simulink model "ACFT"  (R2025a)
settings: Solver=ode1  StartTime=0.0  StopTime=200  FixedStep=0.01  RelTol=1e-3  EnableMultiTasking=on
model workspace (MAT data in the model file):
  op_trim2 : opcond.OperatingReport (value not decoded)
values from neighbouring files (symbols this model uses):
  alfaf_deg = -1.8    [initACFT_low.m]
  b = 21    [initACFT_low.m]
  c = 2.5    [initACFT_low.m]
  CD0 = 0.0230    (= 0.023)    [initACFT_low.m]
  CD_alpha = 0.1318    [initACFT_low.m]
  CD_elev = 0.0178    [initACFT_low.m]
  CL0 = 0.19    [initACFT_low.m]
  Cl_ail = -0.0516    [initACFT_low.m]
  CL_alpha = 6.1879    [initACFT_low.m]
  CL_AlphaDot = 1.93    [initACFT_low.m]
  Cl_beta = -0.1352    [initACFT_low.m]
  CL_elev = 0.4727    [initACFT_low.m]
  Cl_p = -0.45    [initACFT_low.m]
  CL_q = 4.66    [initACFT_low.m]
  Cl_r = 0.100    (= 0.1)    [initACFT_low.m]
  Cl_rud = 0.0289    [initACFT_low.m]
  Cm0 = 0.0133    [initACFT_low.m]
  Cm_alpha = -2.0168    [initACFT_low.m]
  Cm_AlphaDot = -6.76    [initACFT_low.m]
  Cm_elev = -1.6788    [initACFT_low.m]
  Cm_q = -36.3    [initACFT_low.m]
  Cn_ail = -6.3025e-4    (= -0.00063025)    [initACFT_low.m]
  Cn_beta = 0.1209    [initACFT_low.m]
  Cn_p = -0.114    [initACFT_low.m]
  Cn_r = -0.30    (= -0.3)    [initACFT_low.m]
  Cn_rud = -0.1020    (= -0.102)    [initACFT_low.m]
  CY_ail = 0    [initACFT_low.m]
  CY_beta = -1.1803    [initACFT_low.m]
  CY_p = 0.3    [initACFT_low.m]
  CY_r = 0.910    (= 0.91)    [initACFT_low.m]
  CY_rud = 0.4016    [initACFT_low.m]
  g = 9.80665    [initACFT_low.m]
  Inertia = [Ixx 0 -Ixz; 0 Iyy 0; -Ixz 0 Izz]    [initACFT_low.m]
  nrho = 0.75    [initACFT_low.m]
  nv = 0    [initACFT_low.m]
  rho_reference_kgpm3 = 1.225    [initACFT_low.m]
  S = 45    [initACFT_low.m]
  Tmax = 68000    [initACFT_low.m]
  V_reference_mps = 200    [initACFT_low.m]
  xf_m = -3.8    [initACFT_low.m]
  y_cg = 0    [initACFT_low.m]
  z_cg = -0.4    [initACFT_low.m]
  zf_m = -0.6    [initACFT_low.m]
undefined symbols (not defined in the file or in its folder): EqM
settings Model: PacingRate=0.890000  Creator=bruno  LastModifiedBy=best
settings SolverCC: AlgebraicLoopSolver=TrustRegion
settings DataIOCC: ExternalInput=getinputstruct(op_trim2)  InitialState=getstatestruct(op_trim2)  LoadExternalInput=on  LoadInitialState=on  ReturnWorkspaceOutputs=off
settings OptimizationCC: LifeSpan=inf
settings DebuggingCC: UnconnectedInputMsg=warning  UnconnectedOutputMsg=warning  UnconnectedLineMsg=warning  SFUnexpectedBacktrackingDiag=warning  SFNoUnconditionalDefaultTransitionDiag=warning  ArithmeticOperatorsInVariantConditions=warning
settings ModelReferenceCC: EnableRefExpFcnMdlSchedulingChecks=on
settings SFSimCC: SimUseLocalCustomCode=off  CustomCodeUndefinedFunction=UseInterfaceOnly
settings RTWCC: RTWUseLocalCustomCode=off  GPUComputeCapability=3.5
settings CodeAppCC: StateflowObjectComments=on
settings GRTTargetCC: TargetLangStandard=C89/C90 (ANSI)
settings ConfigComp: CovMetricSettings=dw  CovSaveCumulativeToWorkspaceVar=on  CovSaveSingleToWorkspaceVar=on  CovExternalEMLEnable=off

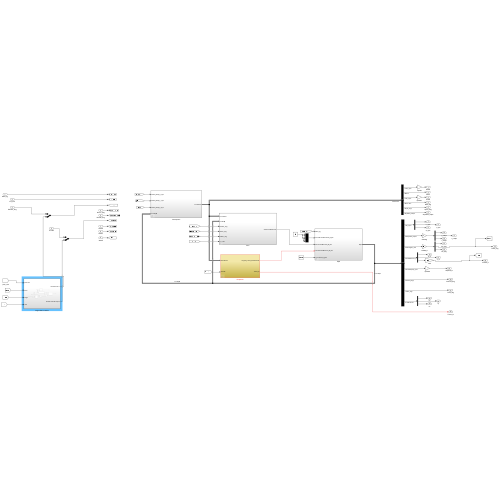
[thumbnail: Simulink's stored preview of the top-level diagram]
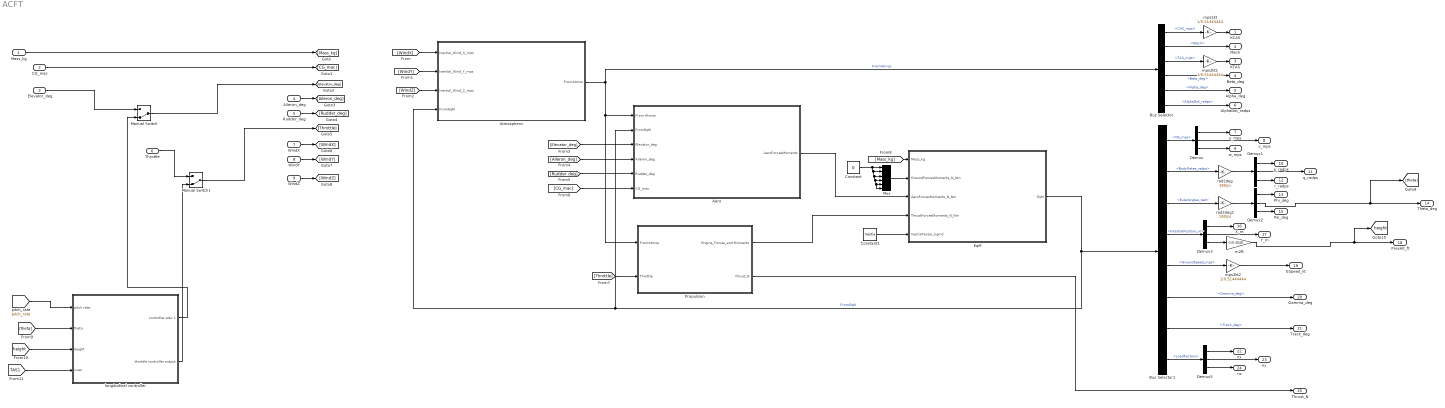
== system ACFT ==
  Mass_kg : Inport  OutDataTypeStr=double
  CG_mac : Inport  Port=2  OutDataTypeStr=double
  Elevator_deg : Inport  Port=3  OutDataTypeStr=double
  Aileron_deg : Inport  Port=4  OutDataTypeStr=double
  Rudder_deg : Inport  Port=5  OutDataTypeStr=double
  Throttle : Inport  Port=6  OutDataTypeStr=double
  WindX : Inport  Port=7  OutDataTypeStr=double
  WindY : Inport  Port=8  OutDataTypeStr=double
  WindZ : Inport  Port=9  OutDataTypeStr=double
  Aero : Subsystem  AncestorBlock=Aerodynamic/Aero
  Atmospheric : Subsystem  AncestorBlock=Atmospheric/Atmospheric
  Bus Selector : BusSelector  OutputSignals=CAS_mps,Mach,TAS_mps,Beta_deg,Alpha_deg,AlphaDot_radps
  Bus Selector1 : BusSelector  OutputSignals=VB_mps,BodyRates_radps,EulerAngles_rad,IntertialPosition_m,GroundSpeed_mps,Gamma_deg,Track_deg,LoadFactors
  Constant : Constant  Value=0  OutDataTypeStr=double
  Constant1 : Constant  Value=Inertia  OutDataTypeStr=double
  Demux{,1..3,5} (5 alike) : Demux  Outputs=3
  EqM : Subsystem  AncestorBlock=EqM/EqM
  Manual Switch : ManualSwitch  CurrentSetting=0
  Manual Switch1 : ManualSwitch  CurrentSetting=0
  Mux : Mux  Inputs=6
  Propulsion : Subsystem  AncestorBlock=Propulsion/Propulsion
  longitudinal controller : Subsystem
  m2ft : Gain  Gain=-1/0.3048
  mps2kt : Gain  Gain=1/0.51444444
  mps2kt1 : Gain  Gain=1/0.51444444
  mps2kt2 : Gain  Gain=1/0.51444444
  rad2deg : Gain  Gain=180/pi
  rad2deg1 : Gain  Gain=180/pi
  KCAS : Outport
  Mach : Outport  Port=2
  KTAS : Outport  Port=3
  Beta_deg : Outport  Port=4
  Alpha_deg : Outport  Port=5
  AlphaDot_radps : Outport  Port=6
  u_mps : Outport  Port=7
  v_mps : Outport  Port=8
  w_mps : Outport  Port=9
  p_radps : Outport  Port=10
  q_radps : Outport  Port=11
  r_radps : Outport  Port=12
  Phi_deg : Outport  Port=13
  Theta_deg : Outport  Port=14
  Psi_deg : Outport  Port=15
  X_m : Outport  Port=16
  Y_m : Outport  Port=17
  PresAlt_ft : Outport  Port=18
  GSpeed_kt : Outport  Port=19
  Gamma_deg : Outport  Port=20
  Track_deg : Outport  Port=21
  nx : Outport  Port=22
  ny : Outport  Port=23
  nz : Outport  Port=24
  Thrust_N : Outport  Port=25
  tag scope: height=global
  wires:
  Atmospheric/1(FromAtmos) -> Propulsion/1(FromAtmos), Aero/1(From Atmos), Bus Selector/1  "FromAtmos"
  Aero/1(AeroForcesMoments) -> EqM/3(AeroForcesMoments_N_Nm)
  Propulsion/1(Engine_Forces_and Moments) -> EqM/4(ThrustForcesMoments_N_Nm)
  EqM/1(EqM) -> Aero/2(FromEqM), Atmospheric/4(FromEqM), Bus Selector1/1  "FromEqM"
  Constant/1 -> Mux/6, Mux/5, Mux/4, Mux/3, Mux/2, Mux/1
  Mux/1 -> EqM/2(GroundForcesMoments_N_Nm)
  Constant1/1 -> EqM/5(InertiaTensor_kgm2)
  Mass_kg/1 -> [Mass_kg]
  CG_mac/1 -> [CG_mac]
  Elevator_deg/1 -> Manual Switch/1
  Aileron_deg/1 -> [Aileron_deg]
  Rudder_deg/1 -> [Rudder_deg]
  Throttle/1 -> Manual Switch1/1
  WindX/1 -> [WindX]
  WindY/1 -> [WindY]
  WindZ/1 -> [WindZ]
  [WindX] -> Atmospheric/1(Inertial_Wind_X_mps)
  [WindY] -> Atmospheric/2(Inertial_Wind_Y_mps)
  [WindZ] -> Atmospheric/3(Inertial_Wind_Z_mps)
  [Elevator_deg] -> Aero/3(Elevator_deg)
  [Aileron_deg] -> Aero/4(Aileron_deg)
  [Rudder_deg] -> Aero/5(Rudder_deg)
  [CG_mac] -> Aero/6(CG_mac)
  [Throttle] -> Propulsion/2(Throttle)
  [Mass_kg] -> EqM/1(Mass_kg)
  Propulsion/2(Thrust_N) -> Thrust_N/1
  Bus Selector/1 -> mps2kt/1  "<CAS_mps>"
  mps2kt/1 -> KCAS/1
  Bus Selector/2 -> Mach/1  "<Mach>"
  Bus Selector/3 -> mps2kt1/1  "<TAS_mps>"
  mps2kt1/1 -> KTAS/1
  Bus Selector/4 -> Beta_deg/1  "<Beta_deg>"
  Bus Selector/5 -> Alpha_deg/1  "<Alpha_deg>"
  Bus Selector/6 -> AlphaDot_radps/1  "<AlphaDot_radps>"
  Bus Selector1/1 -> Demux/1  "<VB_mps>"
  Demux/1 -> u_mps/1
  Demux/2 -> v_mps/1
  Demux/3 -> w_mps/1
  Bus Selector1/2 -> rad2deg/1  "<BodyRates_radps>"
  Demux1/1 -> p_radps/1
  Demux1/2 -> q_radps/1
  Demux1/3 -> r_radps/1
  Bus Selector1/3 -> rad2deg1/1  "<EulerAngles_rad>"
  Demux2/1 -> Phi_deg/1
  Demux2/2 -> [theta], Theta_deg/1
  Demux2/3 -> Psi_deg/1
  rad2deg/1 -> Demux1/1
  rad2deg1/1 -> Demux2/1
  Bus Selector1/4 -> Demux3/1  "<IntertialPosition_m>"
  Demux3/1 -> X_m/1
  Demux3/2 -> Y_m/1
  Demux3/3 -> m2ft/1
  m2ft/1 -> [height], PresAlt_ft/1
  Bus Selector1/5 -> mps2kt2/1  "<GroundSpeed_mps>"
  mps2kt2/1 -> GSpeed_kt/1
  Bus Selector1/6 -> Gamma_deg/1  "<Gamma_deg>"
  Bus Selector1/7 -> Track_deg/1  "<Track_deg>"
  Bus Selector1/8 -> Demux5/1  "<LoadFactors>"
  Demux5/1 -> nx/1
  Demux5/2 -> ny/1
  Demux5/3 -> nz/1
  [pitch_rate] -> longitudinal controller/1(pitch rate)
  [theta] -> longitudinal controller/2(theta)
  [height] -> longitudinal controller/3(height)
  [TAS1] -> longitudinal controller/4(vcas)
  longitudinal controller/1(controller elev 1) -> Manual Switch/2
  Manual Switch/1 -> [Elevator_deg]
  longitudinal controller/2(throttle controller output) -> Manual Switch1/2
  Manual Switch1/1 -> [Throttle]

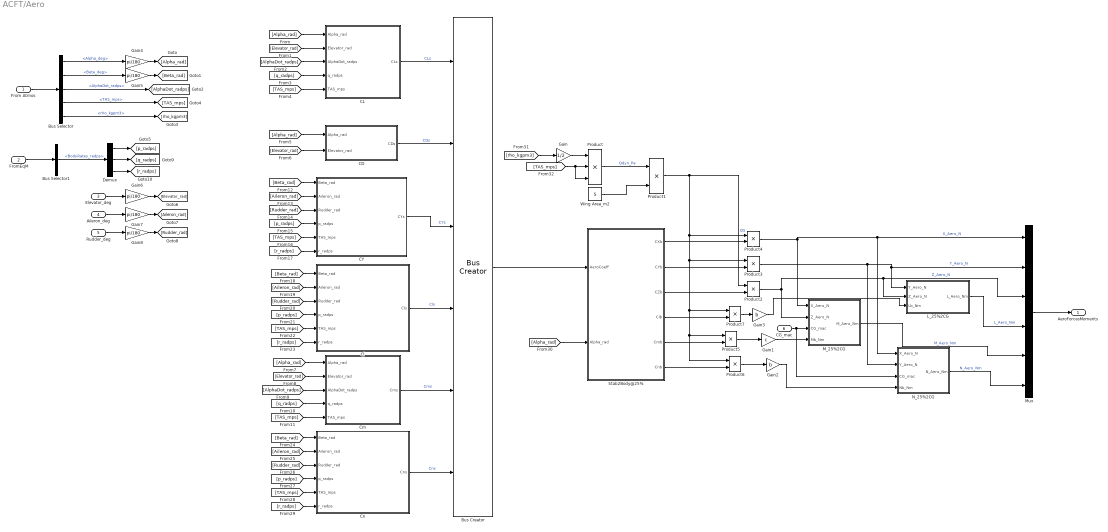
== system ACFT/Aero ==
  From Atmos : Inport
  FromEqM : Inport  Port=2
  Elevator_deg : Inport  Port=3
  Aileron_deg : Inport  Port=4
  Rudder_deg : Inport  Port=5
  CG_mac : Inport  Port=6
  Bus Creator : BusCreator  Inputs=6
  Bus Selector : BusSelector  OutputSignals=Alpha_deg,Beta_deg,AlphaDot_radps,TAS_mps,rho_kgpm3
  Bus Selector1 : BusSelector  OutputSignals=BodyRates_radps
  CD : Subsystem
  CL : Subsystem
  CY : Subsystem
  Cl : Subsystem
  Cm : Subsystem
  Cn : Subsystem
  Demux : Demux  Outputs=3
  Gain : Gain  Gain=1/2
  Gain1 : Gain  Gain=c
  Gain2 : Gain  Gain=b
  Gain3 : Gain  Gain=b
  Gain{4..8} (5 alike) : Gain  Gain=pi/180
  L_25%2CG : Subsystem
  M_25%2CG : Subsystem
  Mux : Mux  Inputs=6
  N_25%2CG : Subsystem
  Product : Product  Inputs=3
  Product{1..7} (7 alike) : Product
  Stab2Body@25% : Subsystem
  Wing Area_m2 : Constant  Value=S
  AeroForcesMoments : Outport
  wires:
  Bus Selector/5 -> [rho_kgpm3]  "<rho_kgpm3>"
  Bus Selector/4 -> [TAS_mps]  "<TAS_mps>"
  N_25%2CG/1(N_Aero_Nm) -> Mux/6  "N_Aero_Nm"
  Product/1 -> Product1/1  "Qdyn_Pa"
  [Aileron_rad] -> Cn/2(Aileron_rad)
  [p_radps] -> Cn/4(p_radps)
  Product5/1 -> Gain1/1
  [q_radps] -> Cm/4(q_radps)
  [AlphaDot_radps] -> Cm/3(AlphaDot_radps)
  CG_mac/1 -> M_25%2CG/3(CG_mac), N_25%2CG/3(CG_mac)
  Product4/1 -> M_25%2CG/1(X_Aero_N), N_25%2CG/1(X_Aero_N), Mux/1  "X_Aero_N"
  [Alpha_rad] -> Stab2Body@25%/2(Alpha_rad)
  Cn/1(Cns) -> Bus Creator/6  "Cns"
  [TAS_mps] -> Cl/5(TAS_mps)
  CL/1(CLs) -> Bus Creator/1  "CLs"
  L_25%2CG/1(L_Aero_Nm) -> Mux/4  "L_Aero_Nm"
  [Aileron_rad] -> CY/2(Aileron_rad)
  Cm/1(Cms) -> Bus Creator/5  "Cms"
  Gain3/1 -> L_25%2CG/3(Lb_Nm)
  Product6/1 -> Gain2/1
  M_25%2CG/1(M_Aero_Nm) -> Mux/5  "M_Aero_Nm"
  CY/1(CYs) -> Bus Creator/3  "CYs"
  [Rudder_rad] -> Cl/3(Rudder_rad)
  [r_radps] -> Cl/6(r_radps)
  Stab2Body@25%/5(Cmb) -> Product5/2
  Gain/1 -> Product/1
  [TAS_mps] -> Cm/5(TAS_mps)
  Stab2Body@25%/3(CZb) -> Product2/2
  [TAS_mps] -> Product/2, Product/3
  [TAS_mps] -> CY/5(TAS_mps)
  Product3/1 -> N_25%2CG/2(Y_Aero_N), L_25%2CG/1(Y_Aero_N), Mux/2  "Y_Aero_N"
  [Aileron_rad] -> Cl/2(Aileron_rad)
  [rho_kgpm3] -> Gain/1
  Product7/1 -> Gain3/1
  Stab2Body@25%/4(Clb) -> Product7/2
  [Rudder_rad] -> Cn/3(Rudder_rad)
  Bus Creator/1 -> Stab2Body@25%/1(AeroCoeff)
  [r_radps] -> Cn/6(r_radps)
  Product2/1 -> M_25%2CG/2(Z_Aero_N), L_25%2CG/2(Z_Aero_N), Mux/3  "Z_Aero_N"
  CD/1(CDs) -> Bus Creator/2  "CDs"
  [TAS_mps] -> Cn/5(TAS_mps)
  Stab2Body@25%/6(Cnb) -> Product6/2
  Product1/1 -> Product4/1, Product5/1, Product6/1, Product7/1, Product3/1, Product2/1  "QS"
  Gain2/1 -> N_25%2CG/4(Nb_Nm)
  Stab2Body@25%/1(CXb) -> Product4/2
  Cl/1(Cls) -> Bus Creator/4  "Cls"
  Wing Area_m2/1 -> Product1/2
  [r_radps] -> CY/6(r_radps)
  [Beta_rad] -> CY/1(Beta_rad)
  [Rudder_rad] -> CY/3(Rudder_rad)
  [Beta_rad] -> Cn/1(Beta_rad)
  [Beta_rad] -> Cl/1(Beta_rad)
  Gain1/1 -> M_25%2CG/4(Mb_Nm)
  [p_radps] -> Cl/4(p_radps)
  Stab2Body@25%/2(CYb) -> Product3/2
  [p_radps] -> CY/4(p_radps)
  Mux/1 -> AeroForcesMoments/1
  Gain5/1 -> [Beta_rad]
  Gain4/1 -> [Alpha_rad]
  Rudder_deg/1 -> Gain8/1
  Bus Selector/3 -> [AlphaDot_radps]  "<AlphaDot_radps>"
  [Elevator_rad] -> Cm/2(Elevator_rad)
  [Alpha_rad] -> Cm/1(Alpha_rad)
  [Elevator_rad] -> CL/2(Elevator_rad)
  Elevator_deg/1 -> Gain6/1
  [Alpha_rad] -> CL/1(Alpha_rad)
  [Elevator_rad] -> CD/2(Elevator_rad)
  Gain8/1 -> [Rudder_rad]
  [Alpha_rad] -> CD/1(Alpha_rad)
  [q_radps] -> CL/4(q_radps)
  Bus Selector/2 -> Gain5/1  "<Beta_deg>"
  Gain7/1 -> [Aileron_rad]
  Aileron_deg/1 -> Gain7/1
  Demux/2 -> [q_radps]
  Demux/1 -> [p_radps]
  Gain6/1 -> [Elevator_rad]
  Demux/3 -> [r_radps]
  [TAS_mps] -> CL/5(TAS_mps)
  [AlphaDot_radps] -> CL/3(AlphaDot_radps)
  From Atmos/1 -> Bus Selector/1
  Bus Selector/1 -> Gain4/1  "<Alpha_deg>"
  FromEqM/1 -> Bus Selector1/1
  Bus Selector1/1 -> Demux/1  "<BodyRates_radps>"

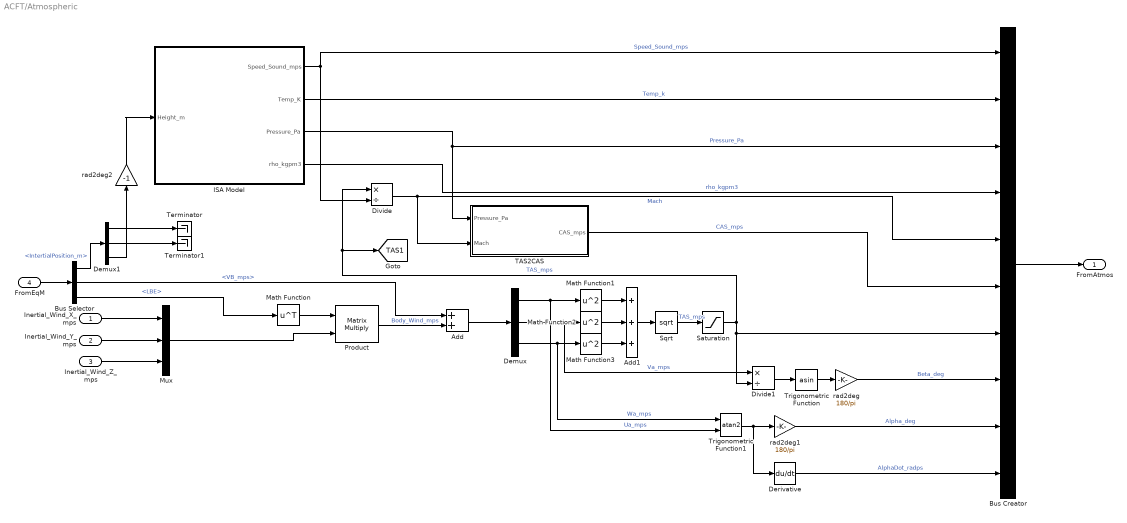
== system ACFT/Atmospheric ==
  Inertial_Wind_X_mps : Inport
  Inertial_Wind_Y_mps : Inport  Port=2
  Inertial_Wind_Z_mps : Inport  Port=3
  FromEqM : Inport  Port=4
  Add : Sum
  Add1 : Sum  Inputs=+++
  Bus Creator : BusCreator  Inputs=10
  Bus Selector : BusSelector  OutputSignals=IntertialPosition_m,VB_mps,LBE
  Demux : Demux  Outputs=3
  Demux1 : Demux  Outputs=3
  Derivative : Derivative
  Divide : Product  Inputs=*/
  Divide1 : Product  Inputs=*/
  ISA Model : Subsystem
  Math Function : Math  Operator=transpose  SignedPower=on
  Math Function1 : Math  Operator=square  SignedPower=on
  Math Function2 : Math  Operator=square  SignedPower=on
  Math Function3 : Math  Operator=square  SignedPower=on
  Mux : Mux  Inputs=3
  Product : Product  Multiplication=Matrix(*)
  Saturation : Saturate  UpperLimit=inf  LowerLimit=1
  Sqrt : Sqrt
  TAS2CAS : Subsystem
  Terminator : Terminator
  Terminator1 : Terminator
  Trigonometric Function : Trigonometry  Operator=asin
  Trigonometric Function1 : Trigonometry  Operator=atan2
  rad2deg : Gain  Gain=180/pi
  rad2deg1 : Gain  Gain=180/pi
  rad2deg2 : Gain  Gain=-1
  FromAtmos : Outport
  tag scope: TAS1=global
  wires:
  rad2deg/1 -> Bus Creator/8  "Beta_deg"
  Math Function3/1 -> Add1/3
  Add1/1 -> Sqrt/1
  Math Function1/1 -> Add1/1
  Demux/2 -> Math Function2/1, Divide1/1  "Va_mps"
  Demux/3 -> Math Function3/1, Trigonometric Function1/1  "Wa_mps"
  Divide1/1 -> Trigonometric Function/1
  Trigonometric Function/1 -> rad2deg/1
  Math Function2/1 -> Add1/2
  Demux/1 -> Math Function1/1, Trigonometric Function1/2  "Ua_mps"
  Add/1 -> Demux/1
  Demux1/3 -> rad2deg2/1
  TAS2CAS/1(CAS_mps) -> Bus Creator/6  "CAS_mps"
  Product/1 -> Add/2  "Body_Wind_mps"
  Mux/1 -> Product/2
  Math Function/1 -> Product/1
  Inertial_Wind_Z_mps/1 -> Mux/3
  Sqrt/1 -> Saturation/1  "TAS_mps"
  FromEqM/1 -> Bus Selector/1
  Divide/1 -> Bus Creator/5, TAS2CAS/2(Mach)  "Mach"
  ISA Model/3(Pressure_Pa) -> Bus Creator/3, TAS2CAS/1(Pressure_Pa)  "Pressure_Pa"
  Inertial_Wind_X_mps/1 -> Mux/1
  ISA Model/2(Temp_K) -> Bus Creator/2  "Temp_k"
  Inertial_Wind_Y_mps/1 -> Mux/2
  ISA Model/1(Speed_Sound_mps) -> Divide/2, Bus Creator/1  "Speed_Sound_mps"
  ISA Model/4(rho_kgpm3) -> Bus Creator/4  "rho_kgpm3"
  rad2deg1/1 -> Bus Creator/9  "Alpha_deg"
  Bus Creator/1 -> FromAtmos/1
  Trigonometric Function1/1 -> rad2deg1/1, Derivative/1
  Derivative/1 -> Bus Creator/10  "AlphaDot_radps"
  Bus Selector/3 -> Math Function/1  "<LBE>"
  Bus Selector/2 -> Add/1  "<VB_mps>"
  Bus Selector/1 -> Demux1/1  "<IntertialPosition_m>"
  Demux1/1 -> Terminator/1
  Demux1/2 -> Terminator1/1
  rad2deg2/1 -> ISA Model/1("Height_m ")
  Saturation/1 -> [TAS1], Divide/1, Bus Creator/7, Divide1/2  "TAS_mps"

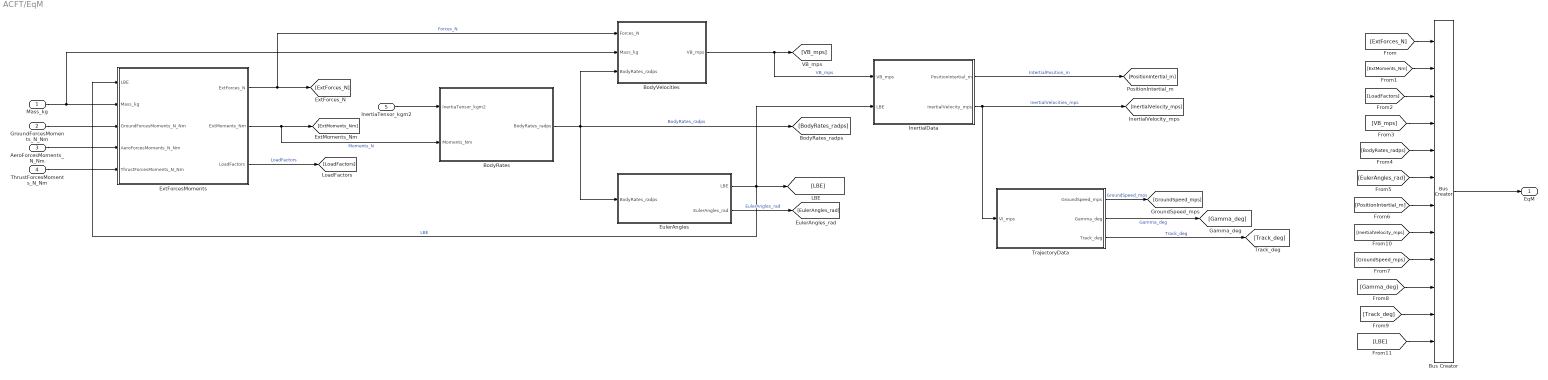
== system ACFT/EqM ==
  Mass_kg : Inport
  GroundForcesMoments_N_Nm : Inport  Port=2
  AeroForcesMoments_N_Nm : Inport  Port=3
  ThrustForcesMoments_N_Nm : Inport  Port=4
  InertiaTensor_kgm2 : Inport  Port=5
  BodyRates : Subsystem
  BodyVelocities : Subsystem
  Bus Creator : BusCreator  Inputs=12
  EulerAngles : Subsystem
  ExtForcesMoments : Subsystem
  InertialData : Subsystem
  TrajectoryData : Subsystem
  EqM : Outport
  wires:
  [PositionIntertial_m] -> Bus Creator/7
  [EulerAngles_rad] -> Bus Creator/6
  [BodyRates_radps] -> Bus Creator/5
  [VB_mps] -> Bus Creator/4
  [ExtForces_N] -> Bus Creator/1
  Bus Creator/1 -> EqM/1
  [Track_deg] -> Bus Creator/11
  [ExtMoments_Nm] -> Bus Creator/2
  [Gamma_deg] -> Bus Creator/10
  [GroundSpeed_mps] -> Bus Creator/9
  TrajectoryData/1(GroundSpeed_mps) -> [GroundSpeed_mps]  "GroundSpeed_mps"
  EulerAngles/2(EulerAngles_rad) -> [EulerAngles_rad]  "EulerAngles_rad"
  TrajectoryData/3(Track_deg) -> [Track_deg]  "Track_deg"
  TrajectoryData/2(Gamma_deg) -> [Gamma_deg]  "Gamma_deg"
  AeroForcesMoments_N_Nm/1 -> ExtForcesMoments/4(AeroForcesMoments_N_Nm)
  ExtForcesMoments/3(LoadFactors) -> [LoadFactors]  "LoadFactors"
  Mass_kg/1 -> ExtForcesMoments/2(Mass_kg), BodyVelocities/2(Mass_kg)
  ExtForcesMoments/1(ExtForces_N) -> BodyVelocities/1(Forces_N), [ExtForces_N]  "Forces_N"
  BodyVelocities/1(VB_mps) -> InertialData/1(VB_mps), [VB_mps]  "VB_mps"
  EulerAngles/1(LBE) -> [LBE], ExtForcesMoments/1(LBE), InertialData/2(LBE)  "LBE"
  GroundForcesMoments_N_Nm/1 -> ExtForcesMoments/3(GroundForcesMoments_N_Nm)
  ThrustForcesMoments_N_Nm/1 -> ExtForcesMoments/5(ThrustForcesMoments_N_Nm)
  BodyRates/1(BodyRates_radps) -> BodyVelocities/3(BodyRates_radps), EulerAngles/1(BodyRates_radps), [BodyRates_radps]  "BodyRates_radps"
  InertiaTensor_kgm2/1 -> BodyRates/1(InertiaTensor_kgm2)
  ExtForcesMoments/2(ExtMoments_Nm) -> BodyRates/2(Moments_Nm), [ExtMoments_Nm]  "Moments_N"
  [InertialVelocity_mps] -> Bus Creator/8
  [LoadFactors] -> Bus Creator/3
  InertialData/2(InertialVelocity_mps) -> TrajectoryData/1(VI_mps), [InertialVelocity_mps]  "InertialVelocities_mps"
  InertialData/1(PositionIntertial_m) -> [PositionIntertial_m]  "IntertialPosition_m"
  [LBE] -> Bus Creator/12

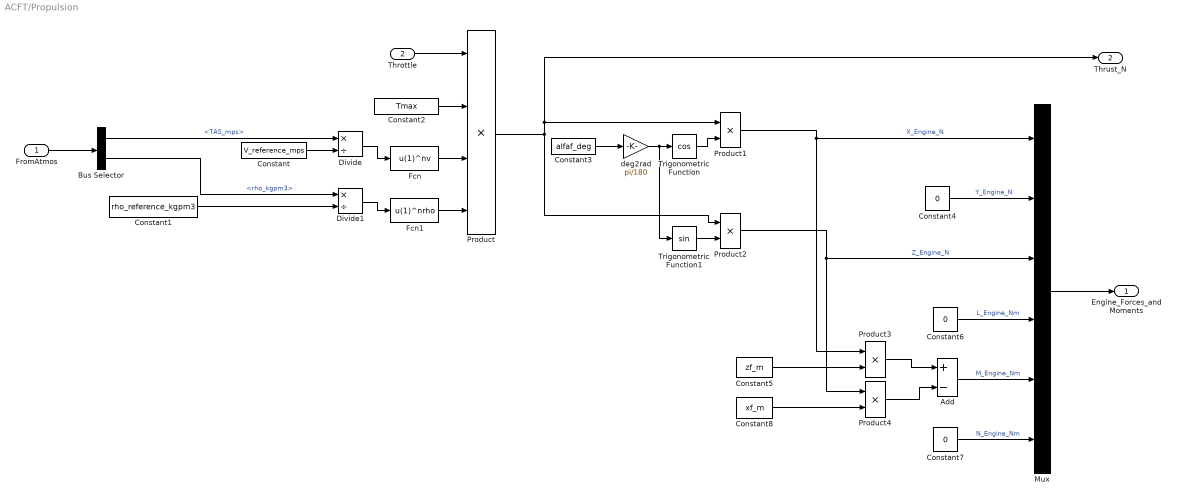
== system ACFT/Propulsion ==
  FromAtmos : Inport
  Throttle : Inport  Port=2
  Add : Sum  Inputs=+-
  Bus Selector : BusSelector  OutputSignals=TAS_mps,rho_kgpm3
  Constant : Constant  Value=V_reference_mps
  Constant1 : Constant  Value=rho_reference_kgpm3
  Constant2 : Constant  Value=Tmax
  Constant3 : Constant  Value=alfaf_deg
  Constant4 : Constant  Value=0
  Constant5 : Constant  Value=zf_m
  Constant6 : Constant  Value=0
  Constant7 : Constant  Value=0
  Constant8 : Constant  Value=xf_m
  Divide : Product  Inputs=*/
  Divide1 : Product  Inputs=*/
  Fcn : Fcn  Expr=u(1)^nv
  Fcn1 : Fcn  Expr=u(1)^nrho
  Mux : Mux  Inputs=6
  Product : Product  Inputs=4
  Product{1..4} (4 alike) : Product
  Trigonometric Function : Trigonometry  Operator=cos
  Trigonometric Function1 : Trigonometry
  deg2rad : Gain  Gain=pi/180
  Engine_Forces_and Moments : Outport
  Thrust_N : Outport  Port=2
  wires:
  Bus Selector/1 -> Divide/1  "<TAS_mps>"
  Add/1 -> Mux/5  "M_Engine_Nm"
  Constant8/1 -> Product4/2
  Constant4/1 -> Mux/2  "Y_Engine_N"
  Trigonometric Function/1 -> Product1/2
  Product1/1 -> Product3/1, Mux/1  "X_Engine_N"
  deg2rad/1 -> Trigonometric Function/1, Trigonometric Function1/1
  Product/1 -> Product1/1, Thrust_N/1, Product2/1
  Mux/1 -> Engine_Forces_and Moments/1
  Product2/1 -> Product4/1, Mux/3  "Z_Engine_N"
  FromAtmos/1 -> Bus Selector/1
  Divide/1 -> Fcn/1
  Constant2/1 -> Product/2
  Fcn/1 -> Product/3
  Bus Selector/2 -> Divide1/1  "<rho_kgpm3>"
  Constant7/1 -> Mux/6  "N_Engine_Nm"
  Fcn1/1 -> Product/4
  Constant6/1 -> Mux/4  "L_Engine_Nm"
  Product4/1 -> Add/2
  Constant3/1 -> deg2rad/1
  Constant5/1 -> Product3/2
  Divide1/1 -> Fcn1/1
  Constant1/1 -> Divide1/2
  Product3/1 -> Add/1
  Constant/1 -> Divide/2
  Throttle/1 -> Product/1
  Trigonometric Function1/1 -> Product2/2

== system ACFT/longitudinal controller ==
  pitch rate : Inport
  theta : Inport  Port=2
  height : Inport  Port=3
  vcas : Inport  Port=4
  Manual Switch : ManualSwitch  CurrentSetting=0
  Manual Switch1 : ManualSwitch  CurrentSetting=0
  Scope : Scope
      settings: ActiveDisplayYMinimum=-90.042313171294722  ActiveDisplayYMaximum=5604.3230575838888
  airspeed_pitchcontrol : Subsystem
  altitude_hold : Subsystem
  commande_pitch : Constant  Value=3
  commanded airspeed : Constant  Value=100
  commanded height : Constant  Value=500
  pitch_attitude_controller : Subsystem
  throttle_control : Subsystem
  controller elev 1 : Outport
  throttle controller output : Outport  Port=2
  wires:
  vcas/1 -> throttle_control/1(vcas), airspeed_pitchcontrol/1(vcas)
  height/1 -> Scope/1, altitude_hold/1(height)
  altitude_hold/1(commanded_pitch) -> Manual Switch/2
  commanded height/1 -> altitude_hold/2(commanded_altitude)
  throttle_control/1(throttle controller output) -> throttle controller output/1
  commanded airspeed/1 -> throttle_control/2(commanded_airspeed), airspeed_pitchcontrol/2(commanded_airspeed)
  commande_pitch/1 -> Manual Switch/1
  airspeed_pitchcontrol/1(commanded_pitch) -> Manual Switch1/1
  pitch rate/1 -> pitch_attitude_controller/1(pitch rate)
  theta/1 -> pitch_attitude_controller/2(theta)
  Manual Switch1/1 -> pitch_attitude_controller/3(commanded_pitch)
  pitch_attitude_controller/1(controller elev 1) -> controller elev 1/1
  Manual Switch/1 -> Manual Switch1/2

== system ACFT/Aero/CD ==
  Alpha_rad : Inport
  Elevator_rad : Inport  Port=2
  Abs : Abs  SaturateOnIntegerOverflow=off
  Abs1 : Abs  SaturateOnIntegerOverflow=off
  Add : Sum  Inputs=+++
  Constant : Constant  Value=CD0
  Gain : Gain  Gain=CD_alpha
  Gain1 : Gain  Gain=CD_elev
  CDs : Outport
  wires:
  Gain/1 -> Add/2
  Alpha_rad/1 -> Abs/1
  Add/1 -> CDs/1
  Elevator_rad/1 -> Abs1/1
  Constant/1 -> Add/1
  Abs/1 -> Gain/1
  Gain1/1 -> Add/3
  Abs1/1 -> Gain1/1

== system ACFT/Aero/CL ==
  Alpha_rad : Inport
  Elevator_rad : Inport  Port=2
  AlphaDot_radps : Inport  Port=3
  q_radps : Inport  Port=4
  TAS_mps : Inport  Port=5
  Add : Sum  Inputs=+++++
  Constant : Constant  Value=CL0
  Divide : Product  Inputs=*/
  Divide1 : Product  Inputs=*/
  Gain : Gain  Gain=CL_alpha
  Gain1 : Gain  Gain=CL_elev
  Gain2 : Gain  Gain=CL_AlphaDot
  Gain3 : Gain  Gain=CL_q
  Gain4 : Gain  Gain=c
  Gain5 : Gain  Gain=2
  Gain6 : Gain  Gain=c
  Gain7 : Gain  Gain=2
  CLs : Outport
  wires:
  AlphaDot_radps/1 -> Gain2/1
  Elevator_rad/1 -> Gain1/1
  q_radps/1 -> Gain3/1
  Gain/1 -> Add/2
  Constant/1 -> Add/1
  Gain1/1 -> Add/3
  Alpha_rad/1 -> Gain/1
  Add/1 -> CLs/1
  Gain3/1 -> Gain4/1
  Gain4/1 -> Divide/1
  TAS_mps/1 -> Gain7/1, Gain5/1
  Gain5/1 -> Divide/2
  Divide/1 -> Add/5
  Gain2/1 -> Gain6/1
  Gain6/1 -> Divide1/1
  Gain7/1 -> Divide1/2
  Divide1/1 -> Add/4

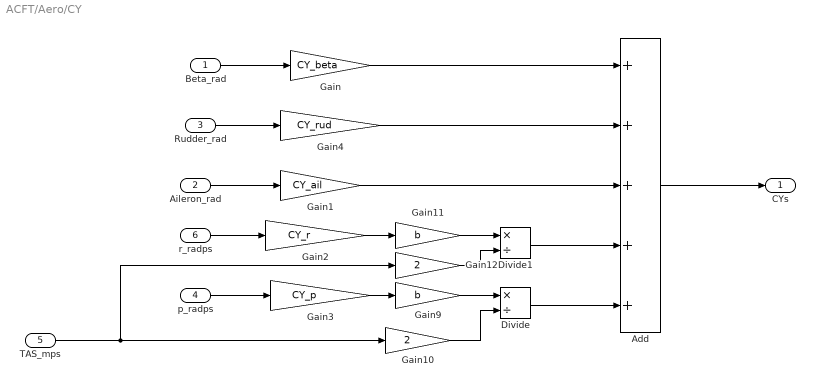
== system ACFT/Aero/CY ==
  Beta_rad : Inport
  Aileron_rad : Inport  Port=2
  Rudder_rad : Inport  Port=3
  p_radps : Inport  Port=4
  TAS_mps : Inport  Port=5
  r_radps : Inport  Port=6
  Add : Sum  Inputs=+++++
  Divide : Product  Inputs=*/
  Divide1 : Product  Inputs=*/
  Gain : Gain  Gain=CY_beta
  Gain1 : Gain  Gain=CY_ail
  Gain10 : Gain  Gain=2
  Gain11 : Gain  Gain=b
  Gain12 : Gain  Gain=2
  Gain2 : Gain  Gain=CY_r
  Gain3 : Gain  Gain=CY_p
  Gain4 : Gain  Gain=CY_rud
  Gain9 : Gain  Gain=b
  CYs : Outport
  wires:
  Aileron_rad/1 -> Gain1/1
  p_radps/1 -> Gain3/1
  Gain3/1 -> Gain9/1
  Beta_rad/1 -> Gain/1
  TAS_mps/1 -> Gain12/1, Gain10/1
  Divide/1 -> Add/5
  Add/1 -> CYs/1
  Gain11/1 -> Divide1/1
  Gain12/1 -> Divide1/2
  Gain10/1 -> Divide/2
  Gain1/1 -> Add/3
  Gain9/1 -> Divide/1
  Gain2/1 -> Gain11/1
  Divide1/1 -> Add/4
  Gain/1 -> Add/1
  Rudder_rad/1 -> Gain4/1
  Gain4/1 -> Add/2
  r_radps/1 -> Gain2/1

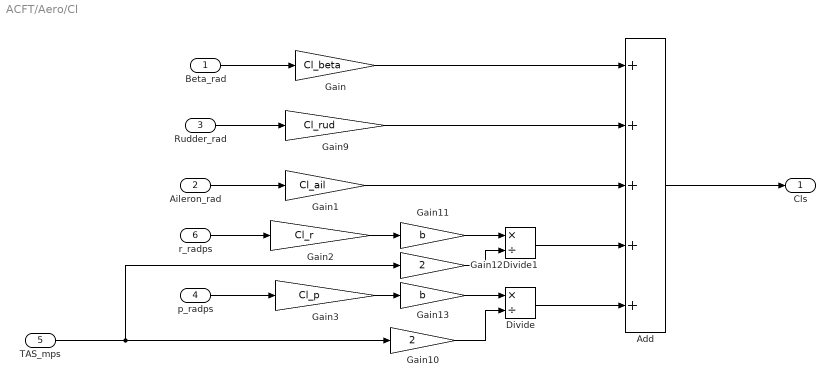
== system ACFT/Aero/Cl ==
  Beta_rad : Inport
  Aileron_rad : Inport  Port=2
  Rudder_rad : Inport  Port=3
  p_radps : Inport  Port=4
  TAS_mps : Inport  Port=5
  r_radps : Inport  Port=6
  Add : Sum  Inputs=+++++
  Divide : Product  Inputs=*/
  Divide1 : Product  Inputs=*/
  Gain : Gain  Gain=Cl_beta
  Gain1 : Gain  Gain=Cl_ail
  Gain10 : Gain  Gain=2
  Gain11 : Gain  Gain=b
  Gain12 : Gain  Gain=2
  Gain13 : Gain  Gain=b
  Gain2 : Gain  Gain=Cl_r
  Gain3 : Gain  Gain=Cl_p
  Gain9 : Gain  Gain=Cl_rud
  Cls : Outport
  wires:
  Aileron_rad/1 -> Gain1/1
  p_radps/1 -> Gain3/1
  Gain3/1 -> Gain13/1
  Beta_rad/1 -> Gain/1
  TAS_mps/1 -> Gain12/1, Gain10/1
  r_radps/1 -> Gain2/1
  Gain1/1 -> Add/3
  Gain11/1 -> Divide1/1
  Gain/1 -> Add/1
  Add/1 -> Cls/1
  Rudder_rad/1 -> Gain9/1
  Gain10/1 -> Divide/2
  Gain12/1 -> Divide1/2
  Gain9/1 -> Add/2
  Gain2/1 -> Gain11/1
  Divide1/1 -> Add/4
  Divide/1 -> Add/5
  Gain13/1 -> Divide/1

== system ACFT/Aero/Cm ==
  Alpha_rad : Inport
  Elevator_rad : Inport  Port=2
  AlphaDot_radps : Inport  Port=3
  q_radps : Inport  Port=4
  TAS_mps : Inport  Port=5
  Add : Sum  Inputs=+++++
  Constant : Constant  Value=Cm0
  Divide : Product  Inputs=*/
  Divide1 : Product  Inputs=*/
  Gain : Gain  Gain=Cm_alpha
  Gain1 : Gain  Gain=Cm_elev
  Gain10 : Gain  Gain=2
  Gain11 : Gain  Gain=c
  Gain12 : Gain  Gain=2
  Gain2 : Gain  Gain=Cm_AlphaDot
  Gain3 : Gain  Gain=Cm_q
  Gain9 : Gain  Gain=c
  Cms : Outport
  wires:
  AlphaDot_radps/1 -> Gain2/1
  Elevator_rad/1 -> Gain1/1
  Gain/1 -> Add/2
  Alpha_rad/1 -> Gain/1
  Add/1 -> Cms/1
  Gain3/1 -> Gain9/1
  Gain9/1 -> Divide/1
  TAS_mps/1 -> Gain12/1, Gain10/1
  q_radps/1 -> Gain3/1
  Constant/1 -> Add/1
  Gain1/1 -> Add/3
  Divide/1 -> Add/5
  Gain2/1 -> Gain11/1
  Gain12/1 -> Divide1/2
  Gain11/1 -> Divide1/1
  Divide1/1 -> Add/4
  Gain10/1 -> Divide/2

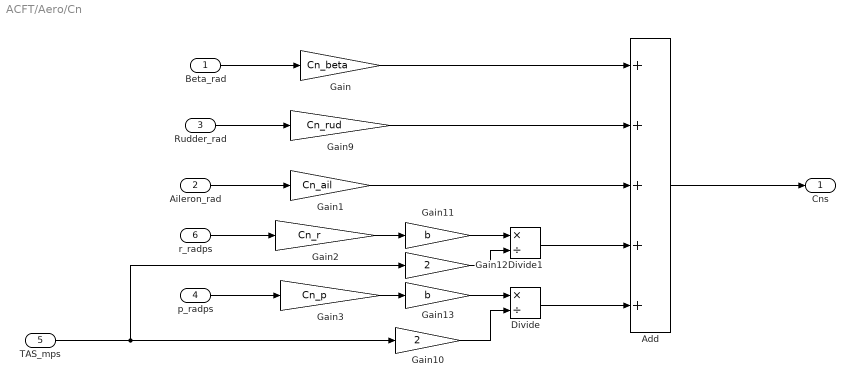
== system ACFT/Aero/Cn ==
  Beta_rad : Inport
  Aileron_rad : Inport  Port=2
  Rudder_rad : Inport  Port=3
  p_radps : Inport  Port=4
  TAS_mps : Inport  Port=5
  r_radps : Inport  Port=6
  Add : Sum  Inputs=+++++
  Divide : Product  Inputs=*/
  Divide1 : Product  Inputs=*/
  Gain : Gain  Gain=Cn_beta
  Gain1 : Gain  Gain=Cn_ail
  Gain10 : Gain  Gain=2
  Gain11 : Gain  Gain=b
  Gain12 : Gain  Gain=2
  Gain13 : Gain  Gain=b
  Gain2 : Gain  Gain=Cn_r
  Gain3 : Gain  Gain=Cn_p
  Gain9 : Gain  Gain=Cn_rud
  Cns : Outport
  wires:
  Gain/1 -> Add/1
  p_radps/1 -> Gain3/1
  Add/1 -> Cns/1
  Gain3/1 -> Gain13/1
  Beta_rad/1 -> Gain/1
  Aileron_rad/1 -> Gain1/1
  TAS_mps/1 -> Gain12/1, Gain10/1
  r_radps/1 -> Gain2/1
  Gain1/1 -> Add/3
  Gain11/1 -> Divide1/1
  Gain12/1 -> Divide1/2
  Rudder_rad/1 -> Gain9/1
  Gain10/1 -> Divide/2
  Gain13/1 -> Divide/1
  Gain2/1 -> Gain11/1
  Gain9/1 -> Add/2
  Divide1/1 -> Add/4
  Divide/1 -> Add/5

== system ACFT/Aero/L_25%2CG ==
  Y_Aero_N : Inport
  Z_Aero_N : Inport  Port=2
  Lb_Nm : Inport  Port=3
  Add : Sum  Inputs=--+
  Product7 : Product
  Product8 : Product
  y_CG_m : Constant  Value=y_cg
  z_CG_m : Constant  Value=z_cg
  L_Aero_Nm : Outport
  wires:
  Z_Aero_N/1 -> Product8/1
  Y_Aero_N/1 -> Product7/1
  y_CG_m/1 -> Product8/2
  Add/1 -> L_Aero_Nm/1  "L_Aero_Nm"
  Lb_Nm/1 -> Add/3
  Product7/1 -> Add/1
  Product8/1 -> Add/2
  z_CG_m/1 -> Product7/2

== system ACFT/Aero/M_25%2CG ==
  X_Aero_N : Inport
  Z_Aero_N : Inport  Port=2
  CG_mac : Inport  Port=3
  Mb_Nm : Inport  Port=4
  Add : Sum  Inputs=-++
  Fcn : Fcn  Expr=(u(1) -0.25)*c
  Product5 : Product
  Product6 : Product
  z_CG_m : Constant  Value=z_cg
  M_Aero_Nm : Outport
  wires:
  z_CG_m/1 -> Product6/2
  Product6/1 -> Add/2
  Add/1 -> M_Aero_Nm/1  "M_Aero_Nm"
  X_Aero_N/1 -> Product6/1
  Z_Aero_N/1 -> Product5/1
  Product5/1 -> Add/1
  Fcn/1 -> Product5/2
  CG_mac/1 -> Fcn/1
  Mb_Nm/1 -> Add/3

== system ACFT/Aero/N_25%2CG ==
  X_Aero_N : Inport
  Y_Aero_N : Inport  Port=2
  CG_mac : Inport  Port=3
  Nb_Nm : Inport  Port=4
  Add : Sum  Inputs=+++
  Fcn : Fcn  Expr=(u(1) -0.25)*c
  Product6 : Product
  Product7 : Product
  y_CG_m : Constant  Value=y_cg
  N_Aero_Nm : Outport
  wires:
  Product7/1 -> Add/2
  y_CG_m/1 -> Product7/2
  Add/1 -> N_Aero_Nm/1  "N_Aero_Nm"
  Nb_Nm/1 -> Add/3
  Fcn/1 -> Product6/2
  Product6/1 -> Add/1
  X_Aero_N/1 -> Product7/1
  CG_mac/1 -> Fcn/1
  Y_Aero_N/1 -> Product6/1

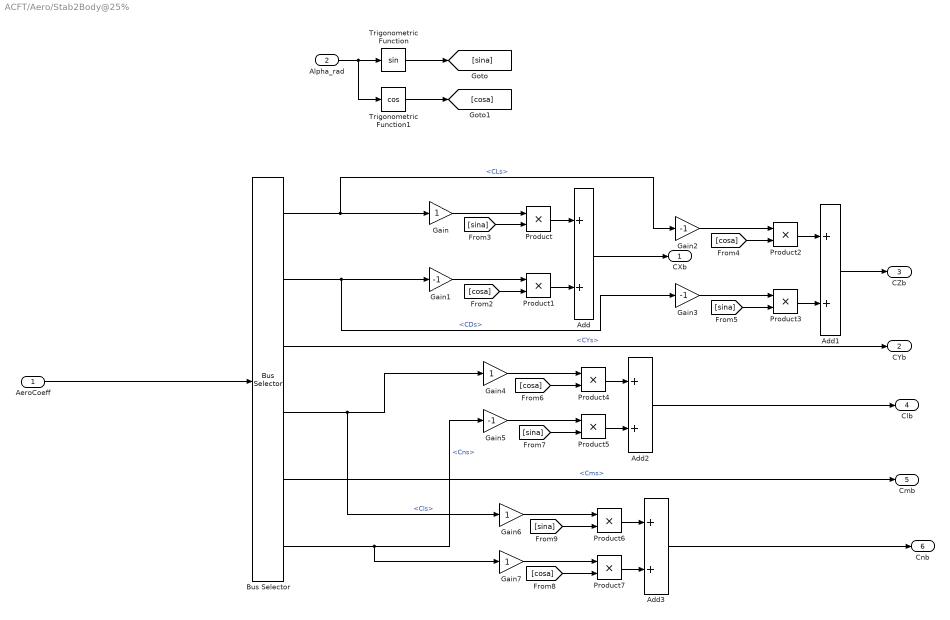
== system ACFT/Aero/Stab2Body@25% ==
  AeroCoeff : Inport
  Alpha_rad : Inport  Port=2
  Add{,1..3} (4 alike) : Sum
  Bus Selector : BusSelector  OutputSignals=CLs,CDs,CYs,Cls,Cms,Cns
  Gain{,4,6..7} (4 alike) : Gain
  Gain{1..3,5} (4 alike) : Gain  Gain=-1
  Product{,1..7} (8 alike) : Product
  Trigonometric Function : Trigonometry
  Trigonometric Function1 : Trigonometry  Operator=cos
  CXb : Outport
  CYb : Outport  Port=2
  CZb : Outport  Port=3
  Clb : Outport  Port=4
  Cmb : Outport  Port=5
  Cnb : Outport  Port=6
  wires:
  AeroCoeff/1 -> Bus Selector/1
  Alpha_rad/1 -> Trigonometric Function1/1, Trigonometric Function/1
  Trigonometric Function/1 -> [sina]
  Trigonometric Function1/1 -> [cosa]
  [sina] -> Product/2
  Bus Selector/1 -> Gain2/1, Gain/1  "<CLs>"
  Gain/1 -> Product/1
  [cosa] -> Product1/2
  Bus Selector/2 -> Gain3/1, Gain1/1  "<CDs>"
  Gain1/1 -> Product1/1
  Product1/1 -> Add/2
  Product/1 -> Add/1
  Add/1 -> CXb/1
  Gain2/1 -> Product2/1
  Gain3/1 -> Product3/1
  Product3/1 -> Add1/2
  Product2/1 -> Add1/1
  Add1/1 -> CZb/1
  [sina] -> Product3/2
  [cosa] -> Product2/2
  Bus Selector/3 -> CYb/1  "<CYs>"
  Bus Selector/5 -> Cmb/1  "<Cms>"
  [cosa] -> Product4/2
  Gain4/1 -> Product4/1
  Gain5/1 -> Product5/1
  Product4/1 -> Add2/1
  Add2/1 -> Clb/1
  Product5/1 -> Add2/2
  Bus Selector/4 -> Gain6/1, Gain4/1  "<Cls>"
  Bus Selector/6 -> Gain7/1, Gain5/1  "<Cns>"
  [sina] -> Product5/2
  [sina] -> Product6/2
  Gain6/1 -> Product6/1
  Gain7/1 -> Product7/1
  Product6/1 -> Add3/1
  Add3/1 -> Cnb/1
  Product7/1 -> Add3/2
  [cosa] -> Product7/2

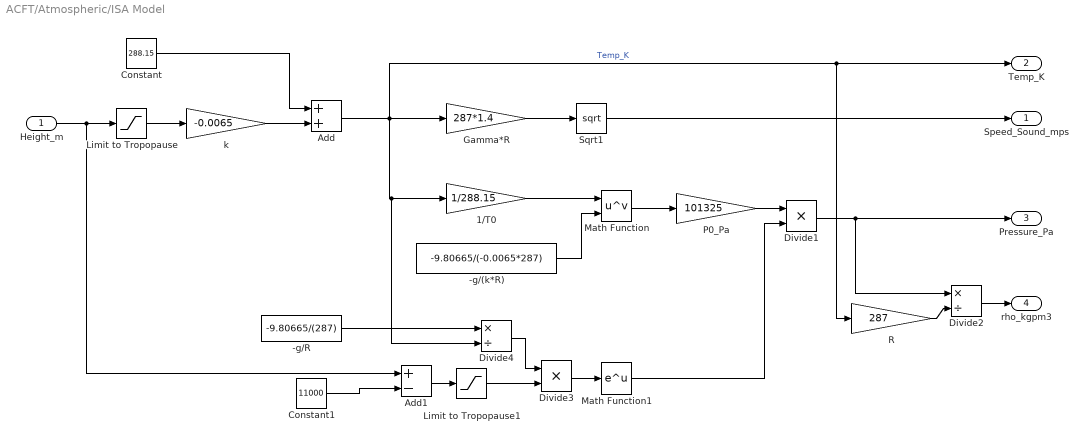
== system ACFT/Atmospheric/ISA Model ==
  "Height_m " : Inport
  -g/(k*R) : Constant  Value=-9.80665/(-0.0065*287)
  -g/R : Constant  Value=-9.80665/(287)
  1/T0 : Gain  Gain=1/288.15
  Add : Sum
  Add1 : Sum  Inputs=+-
  Constant : Constant  Value=288.15
  Constant1 : Constant  Value=11000
  Divide1 : Product  Inputs=**
  Divide2 : Product  Inputs=*/
  Divide3 : Product  Inputs=**
  Divide4 : Product  Inputs=*/
  Gamma*R : Gain  Gain=287*1.4
  Limit to Tropopause : Saturate  UpperLimit=11000  LowerLimit=0
  Limit to Tropopause1 : Saturate  UpperLimit=inf  LowerLimit=0
  Math Function : Math  Operator=pow  SignedPower=on
  Math Function1 : Math  SignedPower=on
  P0_Pa : Gain  Gain=101325
  R : Gain  Gain=287
  Sqrt1 : Sqrt
  k : Gain  Gain=-0.0065
  Speed_Sound_mps : Outport
  Temp_K : Outport  Port=2
  Pressure_Pa : Outport  Port=3
  rho_kgpm3 : Outport  Port=4
  wires:
  Math Function1/1 -> Divide1/2
  Divide3/1 -> Math Function1/1
  Divide4/1 -> Divide3/1
  -g/R/1 -> Divide4/1
  Constant1/1 -> Add1/2
  Divide2/1 -> rho_kgpm3/1
  R/1 -> Divide2/2
  Divide1/1 -> Pressure_Pa/1, Divide2/1
  P0_Pa/1 -> Divide1/1
  Math Function/1 -> P0_Pa/1
  -g/(k*R)/1 -> Math Function/2
  1/T0/1 -> Math Function/1
  Sqrt1/1 -> Speed_Sound_mps/1
  Limit to Tropopause1/1 -> Divide3/2
  Add1/1 -> Limit to Tropopause1/1
  "Height_m "/1 -> Limit to Tropopause/1, Add1/1
  Constant/1 -> Add/1
  k/1 -> Add/2
  Add/1 -> Gamma*R/1, R/1, Temp_K/1, 1/T0/1, Divide4/2  "Temp_K"
  Limit to Tropopause/1 -> k/1
  Gamma*R/1 -> Sqrt1/1

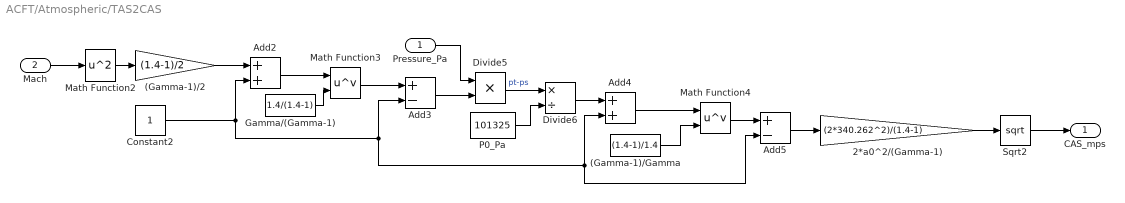
== system ACFT/Atmospheric/TAS2CAS ==
  Pressure_Pa : Inport
  Mach : Inport  Port=2
  (Gamma-1)/2 : Gain  Gain=(1.4-1)/2
  (Gamma-1)/Gamma : Constant  Value=(1.4-1)/1.4
  2*a0^2/(Gamma-1) : Gain  Gain=(2*340.262^2)/(1.4-1)
  Add2 : Sum
  Add3 : Sum  Inputs=+-
  Add4 : Sum
  Add5 : Sum  Inputs=+-
  Constant2 : Constant
  Divide5 : Product  Inputs=**
  Divide6 : Product  Inputs=*/
  Gamma/(Gamma-1) : Constant  Value=1.4/(1.4-1)
  Math Function2 : Math  Operator=square  SignedPower=on
  Math Function3 : Math  Operator=pow  SignedPower=on
  Math Function4 : Math  Operator=pow  SignedPower=on
  P0_Pa : Constant  Value=101325
  Sqrt2 : Sqrt
  CAS_mps : Outport
  wires:
  Sqrt2/1 -> CAS_mps/1
  2*a0^2/(Gamma-1)/1 -> Sqrt2/1
  Add5/1 -> 2*a0^2/(Gamma-1)/1
  Math Function4/1 -> Add5/1
  (Gamma-1)/Gamma/1 -> Math Function4/2
  Add4/1 -> Math Function4/1
  Divide6/1 -> Add4/1
  P0_Pa/1 -> Divide6/2
  Divide5/1 -> Divide6/1  "pt-ps"
  Pressure_Pa/1 -> Divide5/1
  Math Function3/1 -> Add3/1
  Add3/1 -> Divide5/2
  Gamma/(Gamma-1)/1 -> Math Function3/2
  Add2/1 -> Math Function3/1
  Constant2/1 -> Add5/2, Add4/2, Add3/2, Add2/2
  (Gamma-1)/2/1 -> Add2/1
  Mach/1 -> Math Function2/1
  Math Function2/1 -> (Gamma-1)/2/1

== system ACFT/EqM/BodyRates ==
  InertiaTensor_kgm2 : Inport
  Moments_Nm : Inport  Port=2
  CrossProduct : Subsystem
  Demux : Demux  Outputs=3
  Divide : Product  Inputs=/*  Multiplication=Matrix(*)
  Mux : Mux  Inputs=3
  Product : Product  Multiplication=Matrix(*)
  Scope : Scope
      settings: ActiveDisplayYMinimum=-0.33667682832897355  ActiveDisplayYMaximum=0.20770950013646747  DataLoggingVariableName=ScopeData4
  Sum : Sum  Inputs=|-+
  p_radps : Integrator  ContinuousStateAttributes='p_radps'
  q_radps : Integrator  ContinuousStateAttributes='q_radps'
  r_radps : Integrator  ContinuousStateAttributes='r_radps'
  BodyRates_radps : Outport
  tag scope: pitch_rate=global
  wires:
  Divide/1 -> Demux/1
  Demux/2 -> q_radps/1
  Demux/3 -> r_radps/1
  Demux/1 -> p_radps/1
  InertiaTensor_kgm2/1 -> Product/1, Divide/1
  q_radps/1 -> [pitch_rate], Scope/1, Mux/2  "q_radps"
  CrossProduct/1(C) -> Sum/1
  Moments_Nm/1 -> Sum/2
  Product/1 -> CrossProduct/2(B)
  p_radps/1 -> Mux/1  "p_radps"
  Sum/1 -> Divide/2
  Mux/1 -> Product/2, CrossProduct/1(A), BodyRates_radps/1
  r_radps/1 -> Mux/3  "r_radps"

== system ACFT/EqM/BodyVelocities ==
  Forces_N : Inport
  Mass_kg : Inport  Port=2
  BodyRates_radps : Inport  Port=3
  Add : Sum  Inputs=+-
  CrossProduct : Subsystem
  Demux : Demux  Outputs=3
  Divide : Product  Inputs=*/
  Mux : Mux  Inputs=3
  u_mps : Integrator  ContinuousStateAttributes='u_mps'
  v_mps : Integrator  ContinuousStateAttributes='v_mps'
  w_mps : Integrator  ContinuousStateAttributes='w_mps'
  VB_mps : Outport
  wires:
  Mass_kg/1 -> Divide/2
  u_mps/1 -> Mux/1
  Demux/3 -> w_mps/1
  Demux/2 -> v_mps/1
  w_mps/1 -> Mux/3
  v_mps/1 -> Mux/2
  Demux/1 -> u_mps/1
  CrossProduct/1(C) -> Add/2
  BodyRates_radps/1 -> CrossProduct/1(A)
  Mux/1 -> VB_mps/1, CrossProduct/2(B)
  Forces_N/1 -> Divide/1
  Add/1 -> Demux/1  "VB_dot_mps2"
  Divide/1 -> Add/1

== system ACFT/EqM/EulerAngles ==
  BodyRates_radps : Inport
  Demux : Demux  Outputs=3
  EulerRates : Subsystem
  LBE_rotation : Subsystem
  Mux1 : Mux  Inputs=3
  PHI_rad : Integrator  ContinuousStateAttributes='PHI_rad'
  PSI_rad : Integrator  ContinuousStateAttributes='PSI_rad'
  THETA_rad : Integrator  ContinuousStateAttributes='THETA_rad'
  LBE : Outport
  EulerAngles_rad : Outport  Port=2
  wires:
  BodyRates_radps/1 -> EulerRates/1(BodyRates_radps)
  LBE_rotation/1(LBE) -> LBE/1
  EulerRates/1(EulerRates_radsps2) -> Demux/1
  Demux/1 -> PHI_rad/1
  Mux1/1 -> LBE_rotation/1(EulerAngles_rad), EulerAngles_rad/1, EulerRates/2(EulerAngles_rad)
  PSI_rad/1 -> Mux1/3
  THETA_rad/1 -> Mux1/2
  PHI_rad/1 -> Mux1/1
  Demux/3 -> PSI_rad/1
  Demux/2 -> THETA_rad/1

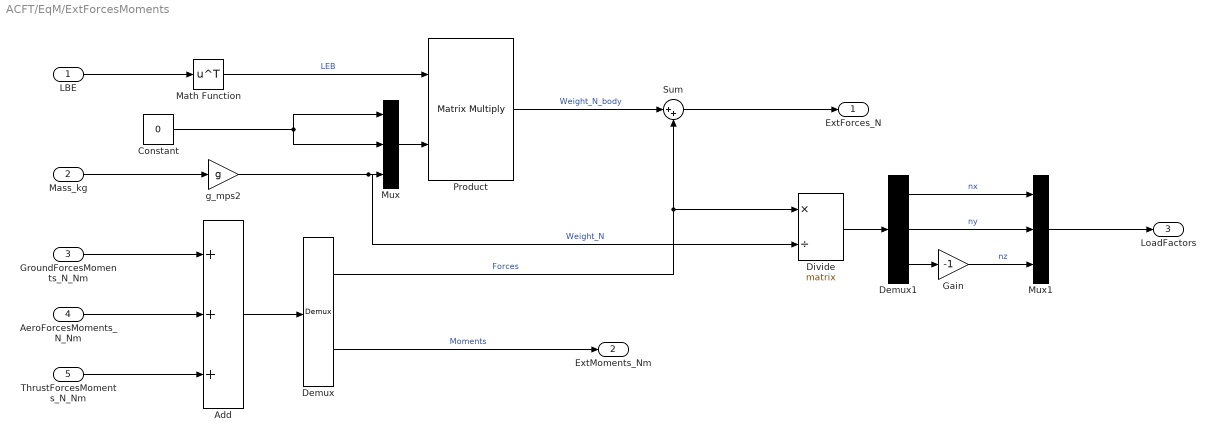
== system ACFT/EqM/ExtForcesMoments ==
  LBE : Inport
  Mass_kg : Inport  Port=2
  GroundForcesMoments_N_Nm : Inport  Port=3
  AeroForcesMoments_N_Nm : Inport  Port=4
  ThrustForcesMoments_N_Nm : Inport  Port=5
  Add : Sum  Inputs=+++
  Constant : Constant  Value=0
  Demux : Demux  Outputs=2
  Demux1 : Demux  Outputs=3
  Divide : Product  Inputs=*/  Multiplication=Matrix(*)
  Gain : Gain  Gain=-1
  Math Function : Math  Operator=transpose  SignedPower=on
  Mux : Mux  Inputs=3
  Mux1 : Mux  Inputs=3
  Product : Product  Multiplication=Matrix(*)
  Sum : Sum  Inputs=|++
  g_mps2 : Gain  Gain=g
  ExtForces_N : Outport
  ExtMoments_Nm : Outport  Port=2
  LoadFactors : Outport  Port=3
  wires:
  Product/1 -> Sum/1  "Weight_N_body"
  Sum/1 -> ExtForces_N/1
  Divide/1 -> Demux1/1
  ThrustForcesMoments_N_Nm/1 -> Add/3
  Mux/1 -> Product/2
  Add/1 -> Demux/1
  LBE/1 -> Math Function/1
  g_mps2/1 -> Mux/3, Divide/2  "Weight_N"
  Mass_kg/1 -> g_mps2/1
  Demux1/1 -> Mux1/1  "nx"
  Demux1/2 -> Mux1/2  "ny"
  AeroForcesMoments_N_Nm/1 -> Add/2
  Mux1/1 -> LoadFactors/1
  Demux1/3 -> Gain/1
  Gain/1 -> Mux1/3  "nz"
  Demux/2 -> ExtMoments_Nm/1  "Moments"
  Constant/1 -> Mux/1, Mux/2
  GroundForcesMoments_N_Nm/1 -> Add/1
  Math Function/1 -> Product/1  "LEB"
  Demux/1 -> Divide/1, Sum/2  "Forces"

== system ACFT/EqM/InertialData ==
  VB_mps : Inport
  LBE : Inport  Port=2
  Demux : Demux  Outputs=3
  Mux : Mux  Inputs=3
  Product : Product  Multiplication=Matrix(*)
  XI_m : Integrator  ContinuousStateAttributes='XI_m'
  YI_m1 : Integrator  ContinuousStateAttributes='YI_m'
  ZI_m : Integrator  ContinuousStateAttributes='ZI_m'
  PositionIntertial_m : Outport
  InertialVelocity_mps : Outport  Port=2
  wires:
  Demux/3 -> ZI_m/1
  Demux/2 -> YI_m1/1
  Demux/1 -> XI_m/1
  Product/1 -> Demux/1, InertialVelocity_mps/1  "VI_mps"
  ZI_m/1 -> Mux/3
  XI_m/1 -> Mux/1
  YI_m1/1 -> Mux/2
  Mux/1 -> PositionIntertial_m/1
  VB_mps/1 -> Product/2
  LBE/1 -> Product/1

== system ACFT/EqM/TrajectoryData ==
  VI_mps : Inport
  Add : Sum
  Demux : Demux  Outputs=3
  Gain : Gain  Gain=-1
  Gain1 : Gain  Gain=180/pi
  Gain2 : Gain  Gain=180/pi
  Math Function : Math  Operator=square  SignedPower=on
  Math Function1 : Math  Operator=square  SignedPower=on
  Sqrt : Sqrt
  Trigonometric Function : Trigonometry  Operator=atan2
  Trigonometric Function1 : Trigonometry  Operator=atan2
  GroundSpeed_mps : Outport
  Gamma_deg : Outport  Port=2
  Track_deg : Outport  Port=3
  wires:
  VI_mps/1 -> Demux/1
  Trigonometric Function1/1 -> Gain2/1
  Gain/1 -> Trigonometric Function/1
  Add/1 -> Sqrt/1
  Demux/1 -> Math Function/1, Trigonometric Function1/2
  Sqrt/1 -> Trigonometric Function/2, GroundSpeed_mps/1
  Demux/2 -> Math Function1/1, Trigonometric Function1/1
  Demux/3 -> Gain/1
  Trigonometric Function/1 -> Gain1/1
  Math Function1/1 -> Add/2
  Math Function/1 -> Add/1
  Gain1/1 -> Gamma_deg/1
  Gain2/1 -> Track_deg/1

== system ACFT/longitudinal controller/airspeed_pitchcontrol ==
  vcas : Inport
  commanded_airspeed : Inport  Port=2
  Gain : Gain  Gain=0.005
  Gain1 : Gain  Gain=8
  Gain2 : Gain
  Integrator : Integrator
  Saturation : Saturate  UpperLimit=10  LowerLimit=-10
  Scope : Scope
      settings: ActiveDisplayYMinimum=10.18072  ActiveDisplayYMaximum=362.78551  DataLoggingVariableName=ScopeData2
  Sum : Sum  Inputs=|+-
  Sum1 : Sum  Inputs=|++
  commandedpitch : Scope
      settings: ActiveDisplayYMinimum=-11  ActiveDisplayYMaximum=-9  DataLoggingVariableName=ScopeData9
  commanded_pitch : Outport
  wires:
  Integrator/1 -> Gain/1
  Sum/1 -> Gain1/1, Integrator/1
  vcas/1 -> Scope/1, Sum/2
  commanded_airspeed/1 -> Sum/1
  Gain1/1 -> Sum1/1
  Saturation/1 -> Gain2/1
  Gain/1 -> Sum1/2
  Sum1/1 -> Saturation/1
  Gain2/1 -> commanded_pitch/1, commandedpitch/1

== system ACFT/longitudinal controller/altitude_hold ==
  height : Inport
  commanded_altitude : Inport  Port=2
  Gain : Gain  Gain=0.1
  Gain2 : Gain  Gain=0.0000009
  Gain3 : Gain  Gain=0.009
  Integrator1 : Integrator
  Saturation1 : Saturate  UpperLimit=10  LowerLimit=-10
  Sum : Sum  Inputs=|+-
  Sum4 : Sum  Inputs=|+++
  commanded_pitch : Outport
  wires:
  Gain2/1 -> Sum4/2
  commanded_altitude/1 -> Sum/1
  Sum/1 -> Gain3/1, Integrator1/1, Gain/1
  height/1 -> Sum/2
  Sum4/1 -> Saturation1/1
  Integrator1/1 -> Gain2/1
  Gain/1 -> Sum4/1
  Gain3/1 -> Sum4/3
  Saturation1/1 -> commanded_pitch/1

== system ACFT/longitudinal controller/pitch_attitude_controller ==
  pitch rate : Inport
  theta : Inport  Port=2
  commanded_pitch : Inport  Port=3
  Constant : Constant  Value=-15
  Gain1 : Gain  Gain=-1
  Integrator : Integrator
  Manual Switch1 : ManualSwitch
  Saturation : Saturate  UpperLimit=30  LowerLimit=-30
  Scope1 : Scope
      settings: ActiveDisplayYMinimum=-36.29542  ActiveDisplayYMaximum=43.71677  DataLoggingVariableName=ScopeData6
  Scope2 : Scope
      settings: ActiveDisplayYMinimum=-12.378807675522561  ActiveDisplayYMaximum=4.3150508529387714
  Sum1 : Sum  Inputs=|+-
  Sum2 : Sum  Inputs=|+-
  Sum3 : Sum  Inputs=|++
  Transfer Fcn3 : TransferFcn  Numerator=[0.9]  Denominator=[0.03 1]
  deriv : Gain
  elevator deflection : Scope
      settings: ActiveDisplayYMinimum=-3.5910668415023821  ActiveDisplayYMaximum=14.088322587469163  DataLoggingVariableName=ScopeData8
  integ : Gain  Gain=0.1
  prop : Gain  Gain=1.2
  controller elev 1 : Outport
  wires:
  Sum2/1 -> prop/1, Integrator/1
  pitch rate/1 -> deriv/1, Scope1/1
  integ/1 -> Sum3/2
  theta/1 -> Scope2/1, Sum2/2
  Integrator/1 -> integ/1
  prop/1 -> Sum3/1
  Sum1/1 -> Gain1/1
  Sum3/1 -> Sum1/1
  Transfer Fcn3/1 -> Manual Switch1/1
  Saturation/1 -> elevator deflection/1, controller elev 1/1
  deriv/1 -> Sum1/2
  Gain1/1 -> Transfer Fcn3/1
  commanded_pitch/1 -> Sum2/1
  Manual Switch1/1 -> Saturation/1
  Constant/1 -> Manual Switch1/2

== system ACFT/longitudinal controller/throttle_control ==
  vcas : Inport
  commanded_airspeed : Inport  Port=2
  Gain : Gain  Gain=0.005
  Gain1 : Gain  Gain=8
  Integrator : Integrator
  Saturation : Saturate  UpperLimit=1  LowerLimit=0
  Sum : Sum  Inputs=|+-
  Sum1 : Sum  Inputs=|++
  throttle position : Scope
      settings: ActiveDisplayYMinimum=0.04854  ActiveDisplayYMaximum=1.10572  DataLoggingVariableName=ScopeData3
  throttle controller output : Outport
  wires:
  commanded_airspeed/1 -> Sum/1
  Saturation/1 -> throttle position/1, throttle controller output/1
  Gain/1 -> Sum1/2
  Gain1/1 -> Sum1/1
  Integrator/1 -> Gain/1
  vcas/1 -> Sum/2
  Sum/1 -> Gain1/1, Integrator/1
  Sum1/1 -> Saturation/1

== system ACFT/EqM/BodyRates/CrossProduct ==
  A : Inport
  B : Inport  Port=2
  Add : Sum  Inputs=+-
  Demux : Demux  Outputs=3
  Demux1 : Demux  Outputs=3
  Mux : Mux  Inputs=3
  Mux1 : Mux  Inputs=3
  Product{,1..5} (6 alike) : Product
  C : Outport
  wires:
  Add/1 -> C/1  "A X B"
  Product2/1 -> Mux/3
  Product/1 -> Mux/1
  Demux/1 -> Product2/1, Product4/1
  Demux1/2 -> Product2/2, Product3/2
  Demux/3 -> Product1/1, Product3/1
  B/1 -> Demux1/1
  Mux1/1 -> Add/2
  Demux/2 -> Product/1, Product5/1
  A/1 -> Demux/1
  Product3/1 -> Mux1/1
  Demux1/1 -> Product1/2, Product5/2
  Mux/1 -> Add/1
  Product5/1 -> Mux1/3
  Product1/1 -> Mux/2
  Demux1/3 -> Product/2, Product4/2
  Product4/1 -> Mux1/2

== system ACFT/EqM/BodyVelocities/CrossProduct ==
  A : Inport
  B : Inport  Port=2
  Add : Sum  Inputs=+-
  Demux : Demux  Outputs=3
  Demux1 : Demux  Outputs=3
  Mux : Mux  Inputs=3
  Mux1 : Mux  Inputs=3
  Product{,1..5} (6 alike) : Product
  C : Outport
  wires:
  Add/1 -> C/1  "A X B"
  Product2/1 -> Mux/3
  Product/1 -> Mux/1
  Demux/1 -> Product2/1, Product4/1
  Demux1/2 -> Product2/2, Product3/2
  Demux/3 -> Product1/1, Product3/1
  B/1 -> Demux1/1
  Mux1/1 -> Add/2
  Demux/2 -> Product/1, Product5/1
  A/1 -> Demux/1
  Product3/1 -> Mux1/1
  Demux1/1 -> Product1/2, Product5/2
  Mux/1 -> Add/1
  Product5/1 -> Mux1/3
  Product1/1 -> Mux/2
  Demux1/3 -> Product/2, Product4/2
  Product4/1 -> Mux1/2

== system ACFT/EqM/EulerAngles/EulerRates ==
  BodyRates_radps : Inport
  EulerAngles_rad : Inport  Port=2
  Abs : Abs  SaturateOnIntegerOverflow=off
  Constant : Constant  Value=0.001
  Demux : Demux  Outputs=3
  Mux : Mux  Inputs=3
  Mux1 : Mux  Inputs=3
  Mux2 : Mux  Inputs=3
  Product : Product
  Relay : Relay  OnSwitchValue=.001  OffSwitchValue=0  OnOutputValue=0  OffOutputValue=1
  Sign : Signum
  Switch : Switch  Criteria=u2 > Threshold  Threshold=0.5  SaturateOnIntegerOverflow=off  InputSameDT=off
  Trigonometric Function : Trigonometry  Operator=sincos
  phidot_radps2 : Fcn  Expr=u(1)+u(2)*u(4)*(u(5)/u(8))+u(3)*u(7)*(u(5)/u(8))
  psidot_radps2 : Fcn  Expr=(u(2)*u(4)+u(3)*u(7))/u(8)
  thetadot_radps2 : Fcn  Expr=u(2)*u(7)-u(3)*u(4)
  EulerRates_radsps2 : Outport
  wires:
  Mux1/1 -> Mux/3
  Trigonometric Function/1 -> Mux/2
  Demux/3 -> Mux1/3
  Constant/1 -> Product/1
  Sign/1 -> Product/2
  Switch/1 -> Mux1/2
  Demux/2 -> Switch/3, Abs/1, Sign/1
  Mux2/1 -> EulerRates_radsps2/1
  psidot_radps2/1 -> Mux2/3
  Product/1 -> Switch/1
  Abs/1 -> Relay/1
  thetadot_radps2/1 -> Mux2/2
  phidot_radps2/1 -> Mux2/1
  BodyRates_radps/1 -> Mux/1
  Relay/1 -> Switch/2
  Demux/1 -> Mux1/1
  Trigonometric Function/2 -> Demux/1
  EulerAngles_rad/1 -> Trigonometric Function/1
  Mux/1 -> psidot_radps2/1, thetadot_radps2/1, phidot_radps2/1

== system ACFT/EqM/EulerAngles/LBE_rotation ==
  note: LBE
  EulerAngles_rad : Inport
  Math Function : Math  Operator=transpose  SignedPower=on
  Mux : Mux  Inputs=2
  Mux2 : Mux  Inputs=9
  Reshape : Reshape  OutputDimensionality=Customize  OutputDimensions=[3,3]
  Trigonometric Function : Trigonometry  Operator=sincos
  phidot_radps1 : Fcn  Expr=u(1)*u(2)*u(6) - u(4)*u(3)
  phidot_radps2 : Fcn  Expr=u(5)*u(6)
  phidot_radps3 : Fcn  Expr=u(6)*u(2)*u(4) + u(1)*u(3)
  phidot_radps4 : Fcn  Expr=u(5)*u(3)
  phidot_radps5 : Fcn  Expr=u(1)*u(2)*u(3) + u(4)*u(6)
  phidot_radps6 : Fcn  Expr=u(4)*u(2)*u(3) -u(1)*u(6)
  phidot_radps7 : Fcn  Expr=-u(2)
  phidot_radps8 : Fcn  Expr=u(1)*u(5)
  phidot_radps9 : Fcn  Expr=u(4)*u(5)
  LBE : Outport
  wires:
  phidot_radps9/1 -> Mux2/9
  phidot_radps8/1 -> Mux2/8
  phidot_radps7/1 -> Mux2/7
  phidot_radps5/1 -> Mux2/5
  phidot_radps6/1 -> Mux2/6
  Mux/1 -> phidot_radps4/1, phidot_radps5/1, phidot_radps6/1, phidot_radps7/1, phidot_radps8/1, phidot_radps9/1, phidot_radps2/1, phidot_radps1/1, phidot_radps3/1
  Trigonometric Function/1 -> Mux/1
  phidot_radps1/1 -> Mux2/2
  phidot_radps2/1 -> Mux2/1
  phidot_radps4/1 -> Mux2/4
  phidot_radps3/1 -> Mux2/3
  Math Function/1 -> LBE/1
  Reshape/1 -> Math Function/1
  Mux2/1 -> Reshape/1
  Trigonometric Function/2 -> Mux/2
  EulerAngles_rad/1 -> Trigonometric Function/1
